simulink model "ZOHx2"  (R2020b)
settings: Solver=VariableStepAuto  StartTime=0.0  StopTime=5  MaxStep=0.05  RelTol=1e-3
libraries: simulink x1
settings Model: Creator=corkep  LastModifiedBy=corkep

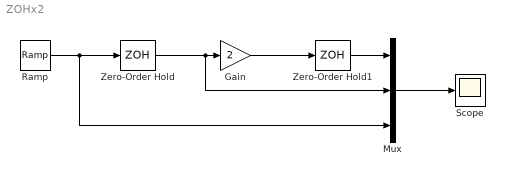
== system ZOHx2 ==
  Gain : Gain  Gain=2
  Mux : Mux  Inputs=3
  Ramp : simulink/Sources/Ramp  slope=1  start=0  InitialOutput=0
  Scope : Scope
  Zero-Order Hold : ZeroOrderHold
  Zero-Order Hold1 : ZeroOrderHold
  wires:
  Ramp/1 -> Zero-Order Hold/1, Mux/3
  Zero-Order Hold/1 -> Mux/2, Gain/1
  Gain/1 -> Zero-Order Hold1/1
  Zero-Order Hold1/1 -> Mux/1
  Mux/1 -> Scope/1
